simulink model "cantoni_combined_matrices_3pools_gates_experiment_splitting_combined"  (R2019b)
settings: Solver=FixedStepDiscrete  StartTime=0.0  StopTime=60*30  FixedStep=1  RelTol=1e-3
undefined symbols (not defined in the file or in its folder): comb_contr, comb_K, comb_plant_disc, comb_plant_disc_p, comb_plant_disc_w, ddelay, Pd, Pd0, Wd
settings Model: Creator=Jacob  LastModifiedBy=bas
settings DataIOCC: ReturnWorkspaceOutputs=off
settings SFSimCC: CustomCodeUndefinedFunction=UseInterfaceOnly

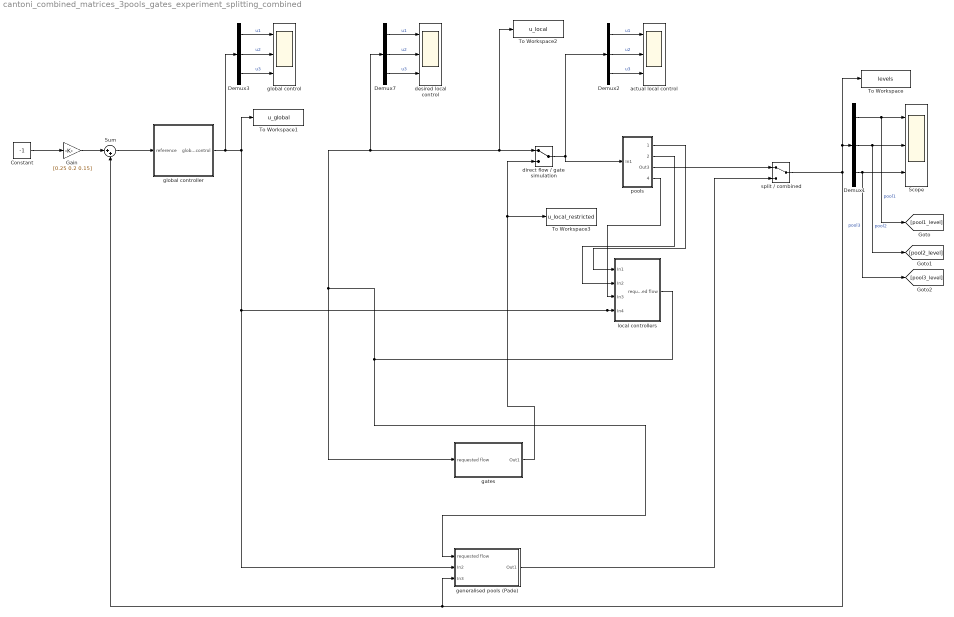
== system cantoni_combined_matrices_3pools_gates_experiment_splitting_combined ==
  Constant : Constant  Value=-1
  Demux{1..3,7} (4 alike) : Demux  Outputs=3
  Gain : Gain  Gain=[0.25 0.2 0.15]
  Scope : Scope  NumInputPorts=3
  Sum : Sum  Inputs=|++
  To Workspace : ToWorkspace  VariableName=levels  SaveFormat=Timeseries  SampleTime=-1
  To Workspace1 : ToWorkspace  VariableName=u_global  SaveFormat=Timeseries  SampleTime=-1
  To Workspace2 : ToWorkspace  VariableName=u_local  SaveFormat=Timeseries  SampleTime=-1
  To Workspace3 : ToWorkspace  VariableName=u_local_restricted  SaveFormat=Timeseries  SampleTime=-1
  actual local control : Scope  NumInputPorts=3
  desired local control : Scope  NumInputPorts=3
  direct flow / gate simulation : ManualSwitch
  gates : Subsystem
  generalised pools (Pade) : Subsystem
  global control : Scope  NumInputPorts=3
  global controller : Subsystem
  local controllers : Subsystem
  pools : Subsystem
  split / combined : ManualSwitch
  wires:
  Constant/1 -> Gain/1
  Gain/1 -> Sum/1
  split / combined/1 -> Sum/2, generalised pools (Pade)/3(In3), Demux1/1, To Workspace/1
  Demux1/1 -> Scope/1, [pool1_level]  "pool1"
  Demux1/2 -> [pool2_level], Scope/2  "pool2"
  Demux1/3 -> [pool3_level], Scope/3  "pool3"
  Demux3/3 -> global control/3  "u3"
  Demux3/2 -> global control/2  "u2"
  Demux3/1 -> global control/1  "u1"
  global controller/1(global_control) -> To Workspace1/1, local controllers/4(In4), generalised pools (Pade)/2(In2), Demux3/1
  Sum/1 -> global controller/1(reference)
  Demux2/3 -> actual local control/3  "u3"
  Demux2/1 -> actual local control/1  "u1"
  Demux2/2 -> actual local control/2  "u2"
  direct flow / gate simulation/1 -> Demux2/1, pools/1(In1)
  Demux7/3 -> desired local control/3  "u3"
  Demux7/2 -> desired local control/2  "u2"
  Demux7/1 -> desired local control/1  "u1"
  pools/3(Out3) -> split / combined/1
  gates/1(Out1) -> To Workspace3/1, direct flow / gate simulation/2
  generalised pools (Pade)/1(Out1) -> split / combined/2
  local controllers/1(requested flow) -> gates/1(requested flow), To Workspace2/1, direct flow / gate simulation/1, Demux7/1, generalised pools (Pade)/1(requested flow)
  pools/1(in_pool1) -> local controllers/1(In1)
  pools/2(in_pool2) -> local controllers/2(In2)
  pools/4(in_pool3) -> local controllers/3(In3)

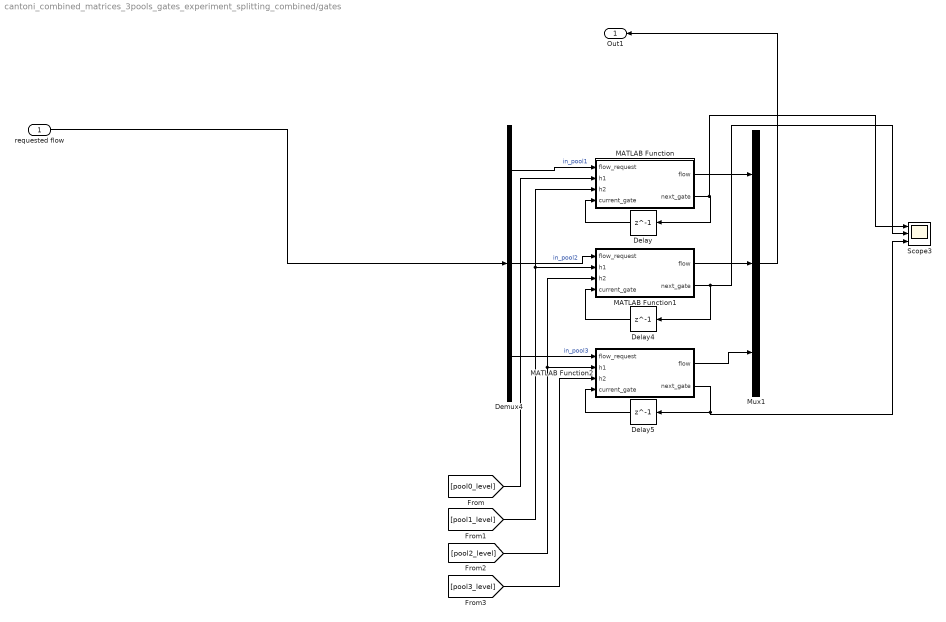
== system cantoni_combined_matrices_3pools_gates_experiment_splitting_combined/gates ==
  requested flow : Inport
  Delay : Delay  DelayLength=1
  Delay4 : Delay  DelayLength=1
  Delay5 : Delay  DelayLength=1
  Demux4 : Demux  Outputs=3
  MATLAB Function : MATLAB Function  TreatAsAtomicUnit=on
  MATLAB Function1 : MATLAB Function  TreatAsAtomicUnit=on
  MATLAB Function2 : MATLAB Function  TreatAsAtomicUnit=on
  Mux1 : Mux  Inputs=3
  Scope3 : Scope  NumInputPorts=3
  Out1 : Outport
  wires:
  Mux1/1 -> Out1/1
  requested flow/1 -> Demux4/1
  [pool2_level] -> MATLAB Function2/2(h1), MATLAB Function1/3(h2)
  Demux4/1 -> MATLAB Function/1(flow_request)  "in_pool1"
  Delay4/1 -> MATLAB Function1/4(current_gate)
  Delay5/1 -> MATLAB Function2/4(current_gate)
  Demux4/2 -> MATLAB Function1/1(flow_request)  "in_pool2"
  MATLAB Function1/2(next_gate) -> Scope3/2, Delay4/1
  [pool3_level] -> MATLAB Function2/3(h2)
  MATLAB Function1/1(flow) -> Mux1/2
  MATLAB Function2/1(flow) -> Mux1/3
  [pool1_level] -> MATLAB Function1/2(h1), MATLAB Function/3(h2)
  Delay/1 -> MATLAB Function/4(current_gate)
  MATLAB Function/1(flow) -> Mux1/1
  Demux4/3 -> MATLAB Function2/1(flow_request)  "in_pool3"
  [pool0_level] -> MATLAB Function/2(h1)
  MATLAB Function2/2(next_gate) -> Scope3/3, Delay5/1
  MATLAB Function/2(next_gate) -> Scope3/1, Delay/1

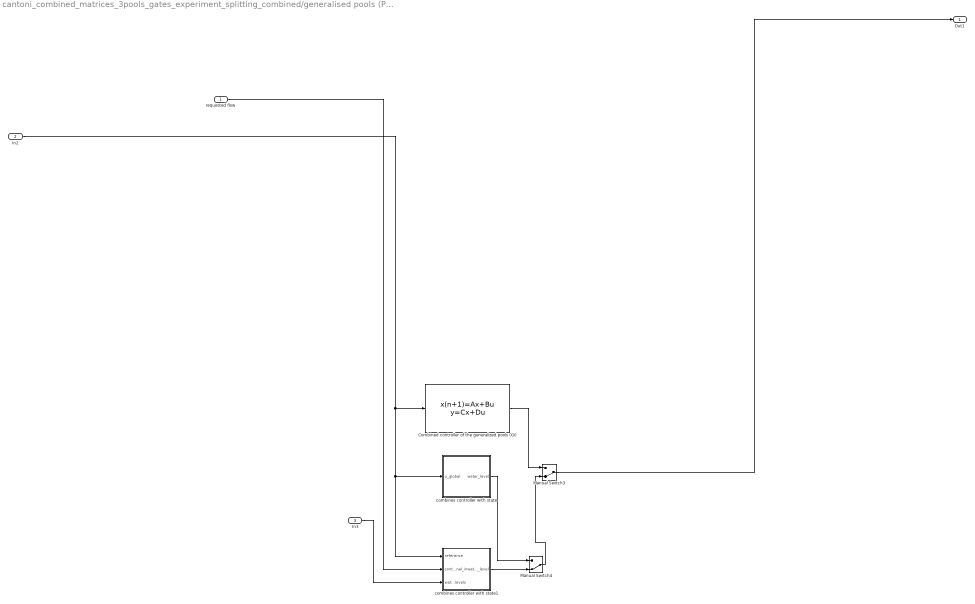
== system cantoni_combined_matrices_3pools_gates_experiment_splitting_combined/generalised pools (Pade) ==
  requested flow : Inport
  In2 : Inport  Port=2
  In3 : Inport  Port=3
  Combined controller of the generalized pools (Gi) : DiscreteStateSpace  A=comb_plant_disc.A  B=comb_plant_disc.B  C=comb_plant_disc.C  D=comb_plant_disc.D  SampleTime=-1
  Manual Switch3 : ManualSwitch  CurrentSetting=0
  Manual Switch4 : ManualSwitch  CurrentSetting=0
  combines controller with state : Subsystem
  combines controller with state1 : Subsystem
  Out1 : Outport
  wires:
  requested flow/1 -> combines controller with state1/2(control_signal_in)
  Combined controller of the generalized pools (Gi)/1 -> Manual Switch3/1
  Manual Switch4/1 -> Manual Switch3/2
  combines controller with state1/1(water_level) -> Manual Switch4/2
  Manual Switch3/1 -> Out1/1
  combines controller with state/1(water_level) -> Manual Switch4/1
  In3/1 -> combines controller with state1/3(water_levels)
  In2/1 -> combines controller with state1/1(reference), combines controller with state/1(u_global), Combined controller of the generalized pools (Gi)/1

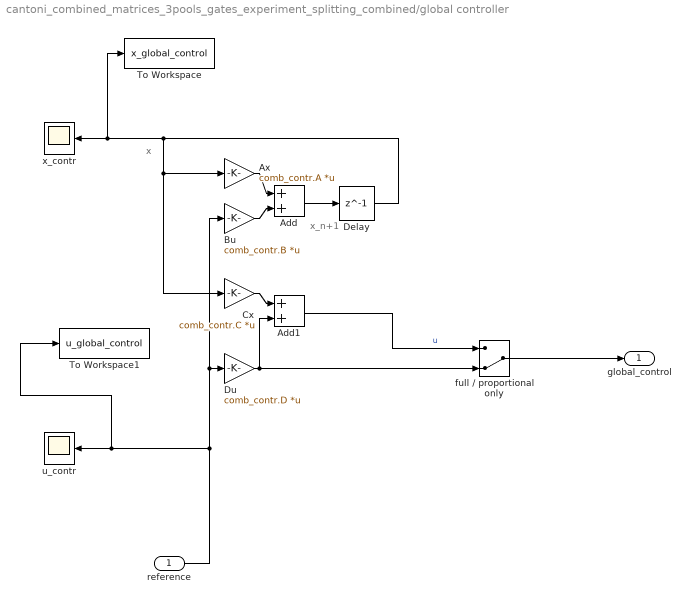
== system cantoni_combined_matrices_3pools_gates_experiment_splitting_combined/global controller ==
  note: x
  note: x_n+1
  reference : Inport
  Add : Sum
  Add1 : Sum
  Ax : Gain  Gain=comb_contr.A  Multiplication=Matrix(K*u)
  Bu : Gain  Gain=comb_contr.B  Multiplication=Matrix(K*u)
  Cx : Gain  Gain=comb_contr.C  Multiplication=Matrix(K*u)
  Delay : Delay  DelayLength=1  InitialCondition=[0;0;0;0;0;0;0;0;0;0;0;0;0;0;0]
  Du : Gain  Gain=comb_contr.D  Multiplication=Matrix(K*u)
  To Workspace : ToWorkspace  VariableName=x_global_control  SaveFormat=Timeseries  SampleTime=-1
  To Workspace1 : ToWorkspace  VariableName=u_global_control  SaveFormat=Timeseries  SampleTime=-1
  full / proportional only : ManualSwitch  CurrentSetting=0
  u_contr : Scope
  x_contr : Scope
  global_control : Outport
  wires:
  Bu/1 -> Add/2
  Cx/1 -> Add1/1
  Add/1 -> Delay/1
  Add1/1 -> full / proportional only/1  "u"
  Ax/1 -> Add/1
  Du/1 -> Add1/2, full / proportional only/2
  full / proportional only/1 -> global_control/1
  reference/1 -> Bu/1, Du/1, To Workspace1/1, u_contr/1
  Delay/1 -> To Workspace/1, x_contr/1, Cx/1, Ax/1

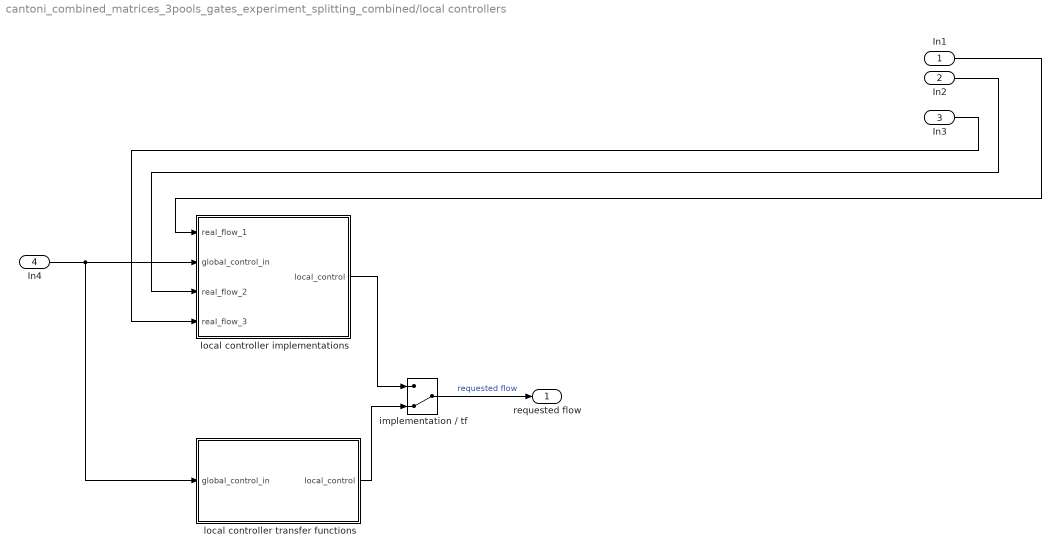
== system cantoni_combined_matrices_3pools_gates_experiment_splitting_combined/local controllers ==
  In1 : Inport
  In2 : Inport  Port=2
  In3 : Inport  Port=3
  In4 : Inport  Port=4
  implementation / tf : ManualSwitch  CurrentSetting=0
  local controller implementations : Subsystem
  local controller transfer functions : Subsystem
  requested flow : Outport
  wires:
  In2/1 -> local controller implementations/3(real_flow_2)
  In3/1 -> local controller implementations/4(real_flow_3)
  implementation / tf/1 -> requested flow/1  "requested flow"
  local controller transfer functions/1(local_control) -> implementation / tf/2
  In1/1 -> local controller implementations/1(real_flow_1)
  In4/1 -> local controller transfer functions/1(global_control_in), local controller implementations/2(global_control_in)
  local controller implementations/1(local_control) -> implementation / tf/1

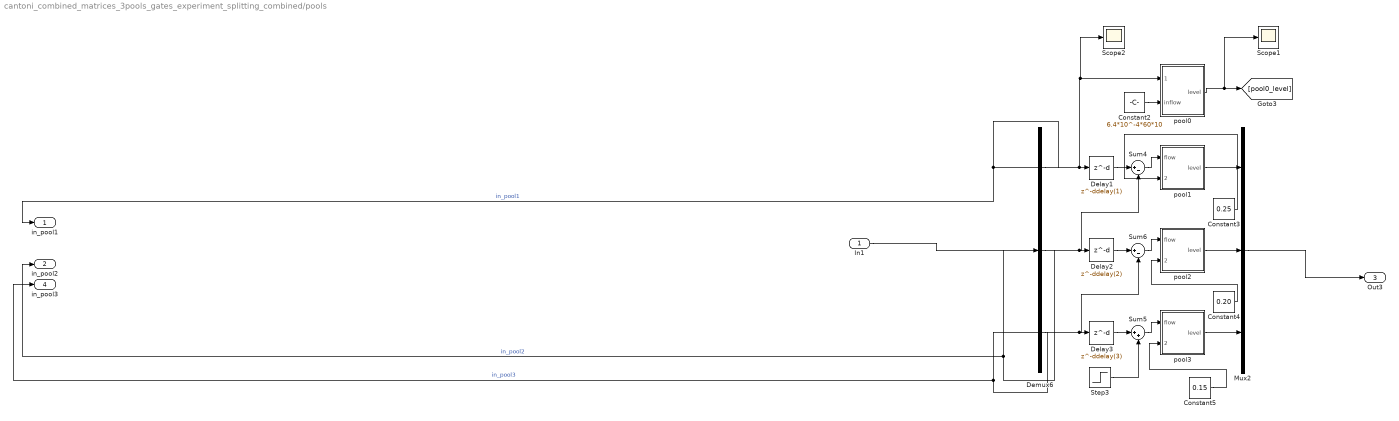
== system cantoni_combined_matrices_3pools_gates_experiment_splitting_combined/pools ==
  In1 : Inport
  Constant2 : Constant  Value=6.4*10^-4*60*10
  Constant3 : Constant  Value=0.25  SampleTime=-1
  Constant4 : Constant  Value=0.20
  Constant5 : Constant  Value=0.15
  Delay1 : Delay  DelayLength=ddelay(1)
  Delay2 : Delay  DelayLength=ddelay(2)
  Delay3 : Delay  DelayLength=ddelay(3)
  Demux6 : Demux  Outputs=3
  Mux2 : Mux  Inputs=3
  Scope1 : Scope
  Scope2 : Scope
  Step3 : Step  Time=100  After=-0.015  SampleTime=0
  Sum4 : Sum  Inputs=|+-
  Sum5 : Sum  Inputs=|++
  Sum6 : Sum  Inputs=|+-
  pool0 : Subsystem
  pool1 : Subsystem
  pool2 : Subsystem
  pool3 : Subsystem
  in_pool1 : Outport
  in_pool2 : Outport  Port=2
  Out3 : Outport  Port=3
  in_pool3 : Outport  Port=4
  wires:
  Mux2/1 -> Out3/1
  pool2/1(level) -> Mux2/2
  Sum6/1 -> pool2/1(flow)
  Sum4/1 -> pool1/1(flow)
  pool3/1(level) -> Mux2/3
  Delay3/1 -> Sum5/1
  pool1/1(level) -> Mux2/1
  Delay2/1 -> Sum6/1
  Delay1/1 -> Sum4/1
  Demux6/2 -> in_pool2/1, Sum4/2, Delay2/1  "in_pool2"
  Constant2/1 -> pool0/2(inflow)
  pool0/1(level) -> Scope1/1, [pool0_level]
  Sum5/1 -> pool3/1(flow)
  Step3/1 -> Sum5/2
  In1/1 -> Demux6/1
  Constant3/1 -> pool1/2("initial_level ")
  Demux6/3 -> in_pool3/1, Sum6/2, Delay3/1  "in_pool3"
  Constant4/1 -> pool2/2(initial_level)
  Constant5/1 -> pool3/2(initial_level)
  Demux6/1 -> in_pool1/1, Scope2/1, pool0/1(outflow), Delay1/1  "in_pool1"

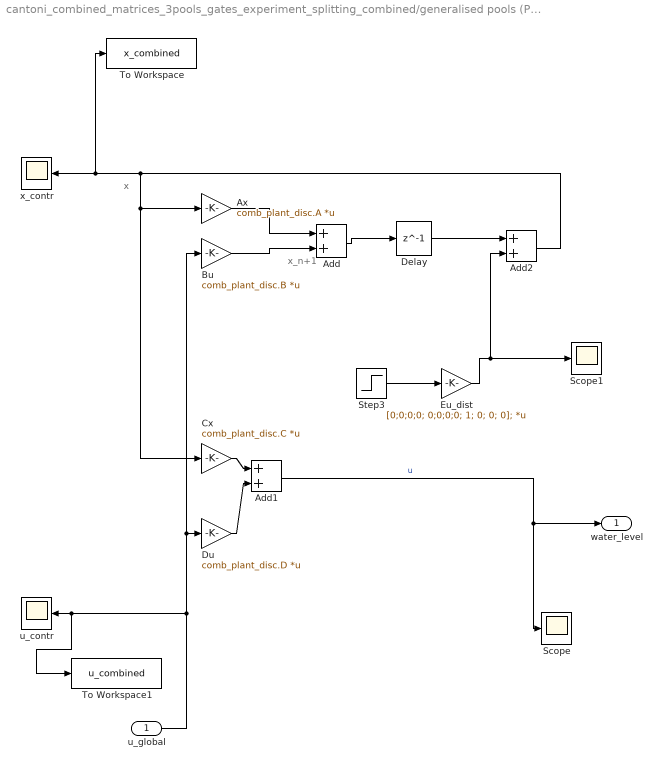
== system cantoni_combined_matrices_3pools_gates_experiment_splitting_combined/generalised pools (Pade)/combines controller with state ==
  note: x
  note: x_n+1
  u_global : Inport
  Add : Sum
  Add1 : Sum
  Add2 : Sum
  Ax : Gain  Gain=comb_plant_disc.A  Multiplication=Matrix(K*u)
  Bu : Gain  Gain=comb_plant_disc.B  Multiplication=Matrix(K*u)
  Cx : Gain  Gain=comb_plant_disc.C  Multiplication=Matrix(K*u)
  Delay : Delay  DelayLength=1  InitialCondition=[0.25;0;0;0;0.20;0;0;0;0.15;0;0;0]
  Du : Gain  Gain=comb_plant_disc.D  Multiplication=Matrix(K*u)
  Eu_dist : Gain  Gain=[0;0;0;0; 0;0;0;0; 1; 0; 0; 0];  Multiplication=Matrix(K*u)
  Scope : Scope
  Scope1 : Scope
  Step3 : Step  Time=100  After=-0.015/0.2279* 1/60  SampleTime=0
  To Workspace : ToWorkspace  VariableName=x_combined  SaveFormat=Timeseries  SampleTime=-1
  To Workspace1 : ToWorkspace  VariableName=u_combined  SaveFormat=Timeseries  SampleTime=-1
  u_contr : Scope
  x_contr : Scope
  water_level : Outport
  wires:
  Bu/1 -> Add/2
  Cx/1 -> Add1/1
  Add/1 -> Delay/1
  Add1/1 -> water_level/1, Scope/1  "u"
  Ax/1 -> Add/1
  Du/1 -> Add1/2
  Add2/1 -> To Workspace/1, x_contr/1, Cx/1, Ax/1
  u_global/1 -> Bu/1, Du/1, To Workspace1/1, u_contr/1
  Step3/1 -> Eu_dist/1
  Eu_dist/1 -> Add2/2, Scope1/1
  Delay/1 -> Add2/1

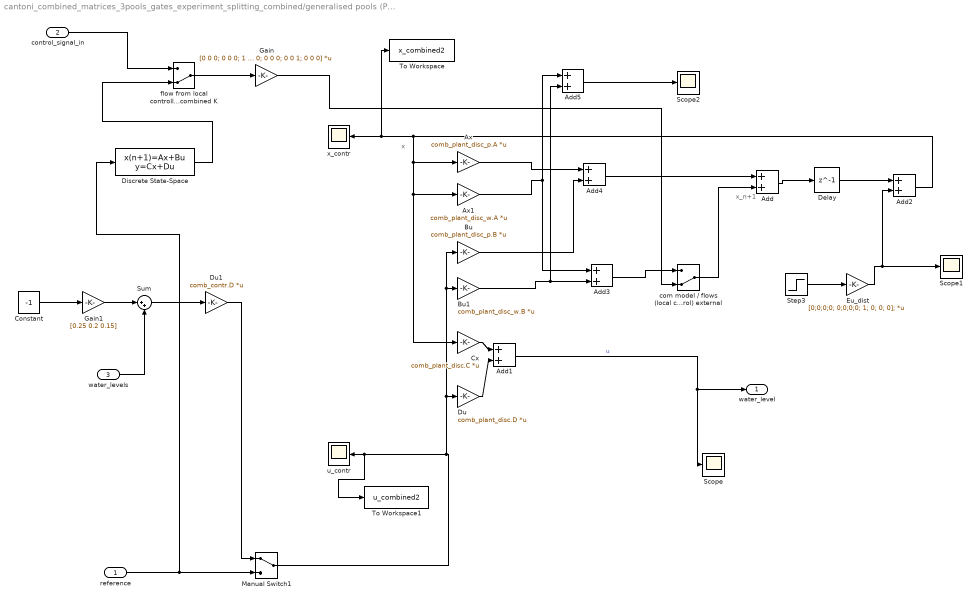
== system cantoni_combined_matrices_3pools_gates_experiment_splitting_combined/generalised pools (Pade)/combines controller with state1 ==
  note: x
  note: x_n+1
  reference : Inport
  control_signal_in : Inport  Port=2
  water_levels : Inport  Port=3
  Add{,1..5} (6 alike) : Sum
  Ax : Gain  Gain=comb_plant_disc_p.A  Multiplication=Matrix(K*u)
  Ax1 : Gain  Gain=comb_plant_disc_w.A  Multiplication=Matrix(K*u)
  Bu : Gain  Gain=comb_plant_disc_p.B  Multiplication=Matrix(K*u)
  Bu1 : Gain  Gain=comb_plant_disc_w.B  Multiplication=Matrix(K*u)
  Constant : Constant  Value=-1
  Cx : Gain  Gain=comb_plant_disc.C  Multiplication=Matrix(K*u)
  Delay : Delay  DelayLength=1  InitialCondition=[0.25;0;0;0;0.20;0;0;0;0.15;0;0;0]
  Discrete State-Space : DiscreteStateSpace  A=comb_K.A  B=comb_K.B  C=comb_K.C  D=comb_K.D  SampleTime=-1
  Du : Gain  Gain=comb_plant_disc.D  Multiplication=Matrix(K*u)
  Du1 : Gain  Gain=comb_contr.D  Multiplication=Matrix(K*u)
  Eu_dist : Gain  Gain=[0;0;0;0; 0;0;0;0; 1; 0; 0; 0];  Multiplication=Matrix(K*u)
  Gain : Gain  Gain=[0 0 0; 0 0 0; 1 0 0; 0 0 0; 0 0 0; 0 0 0; 0 1 0; 0 0 0; 0 0 0; 0 0 0; 0 0 1; 0 0 0]  Multiplication=Matrix(K*u)
  Gain1 : Gain  Gain=[0.25 0.2 0.15]
  Manual Switch1 : ManualSwitch
  Scope : Scope
  Scope1 : Scope
  Scope2 : Scope
  Step3 : Step  Time=100  After=-0.015/0.2279* 1/60  SampleTime=0
  Sum : Sum  Inputs=|++
  To Workspace : ToWorkspace  VariableName=x_combined2  SaveFormat=Timeseries  SampleTime=-1
  To Workspace1 : ToWorkspace  VariableName=u_combined2  SaveFormat=Timeseries  SampleTime=-1
  com model / flows (local control) external : ManualSwitch  CurrentSetting=0
  flow from local controllers / flow from combined K : ManualSwitch  CurrentSetting=0
  u_contr : Scope
  x_contr : Scope
  water_level : Outport
  wires:
  Cx/1 -> Add1/1
  Add/1 -> Delay/1
  Add1/1 -> water_level/1, Scope/1  "u"
  Du/1 -> Add1/2
  Add2/1 -> To Workspace/1, x_contr/1, Ax1/1, Cx/1, Ax/1
  Manual Switch1/1 -> u_contr/1, To Workspace1/1, Bu1/1, Bu/1, Du/1
  Step3/1 -> Eu_dist/1
  Eu_dist/1 -> Add2/2, Scope1/1
  Delay/1 -> Add2/1
  Add4/1 -> Add/1
  Ax/1 -> Add4/1
  Ax1/1 -> Add3/1, Add5/1
  Bu/1 -> Add4/2
  Bu1/1 -> Add5/2, Add3/2
  Add5/1 -> Scope2/1
  control_signal_in/1 -> flow from local controllers / flow from combined K/1
  com model / flows (local control) external/1 -> Add/2
  Add3/1 -> com model / flows (local control) external/1
  Gain/1 -> com model / flows (local control) external/2
  water_levels/1 -> Sum/2
  reference/1 -> Discrete State-Space/1, Manual Switch1/2
  Du1/1 -> Manual Switch1/1
  Gain1/1 -> Sum/1
  Constant/1 -> Gain1/1
  Sum/1 -> Du1/1
  Discrete State-Space/1 -> flow from local controllers / flow from combined K/2
  flow from local controllers / flow from combined K/1 -> Gain/1

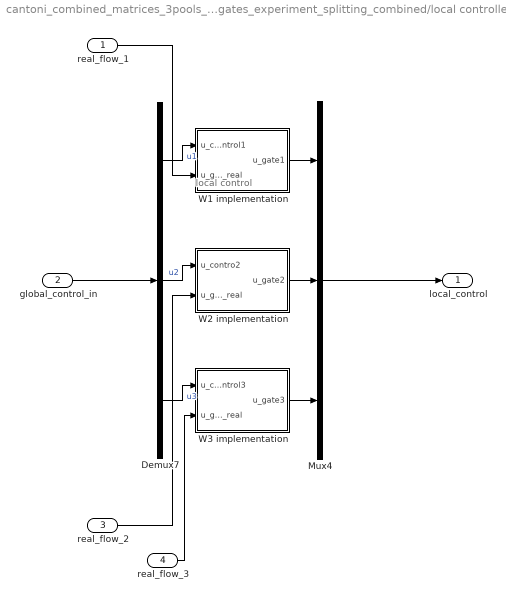
== system cantoni_combined_matrices_3pools_gates_experiment_splitting_combined/local controllers/local controller implementations ==
  note: local control
  real_flow_1 : Inport
  global_control_in : Inport  Port=2
  real_flow_2 : Inport  Port=3
  real_flow_3 : Inport  Port=4
  Demux7 : Demux  Outputs=3
  Mux4 : Mux  Inputs=3
  W1 implementation : Subsystem
  W2 implementation : Subsystem
  W3 implementation : Subsystem
  local_control : Outport
  wires:
  Demux7/1 -> W1 implementation/1(u_control1)  "u1"
  W1 implementation/1(u_gate1) -> Mux4/1
  Demux7/3 -> W3 implementation/1(u_control3)  "u3"
  real_flow_3/1 -> W3 implementation/2(u_gate3_real)
  real_flow_2/1 -> W2 implementation/2(u_gate2_real)
  Demux7/2 -> W2 implementation/1(u_contro2)  "u2"
  global_control_in/1 -> Demux7/1
  Mux4/1 -> local_control/1
  W3 implementation/1(u_gate3) -> Mux4/3
  real_flow_1/1 -> W1 implementation/2(u_gate1_real)
  W2 implementation/1(u_gate2) -> Mux4/2

== system cantoni_combined_matrices_3pools_gates_experiment_splitting_combined/local controllers/local controller transfer functions ==
  global_control_in : Inport
  Demux4 : Demux  Outputs=3
  Mux3 : Mux  Inputs=3
  W1 : DiscreteTransferFcn  Numerator=Wd{1}.Numerator{1}  Denominator=Wd{1}.Denominator{1}
  W2 : DiscreteTransferFcn  Numerator=Wd{2}.Numerator{1}  Denominator=Wd{2}.Denominator{1}
  W3 : DiscreteTransferFcn  Numerator=Wd{3}.Numerator{1}  Denominator=Wd{3}.Denominator{1}
  local_control : Outport
  wires:
  Mux3/1 -> local_control/1
  global_control_in/1 -> Demux4/1
  Demux4/3 -> W3/1  "u3"
  W3/1 -> Mux3/3
  Demux4/2 -> W2/1  "u2"
  W2/1 -> Mux3/2
  W1/1 -> Mux3/1
  Demux4/1 -> W1/1  "u1"

== system cantoni_combined_matrices_3pools_gates_experiment_splitting_combined/pools/pool0 ==
  note: //TODO: remove overflow from pool
  outflow : Inport
  inflow : Inport  Port=2
  Add : Sum  Inputs=-+
  Constant : Constant  Value=0
  Saturation : Saturate  UpperLimit=0.3
  pool1 : DiscreteTransferFcn  Numerator=Pd0.Numerator{1}  Denominator=Pd0.Denominator{1}  InitialStatesSource=Input port
      settings: InputPortMap=u0,p5
  level : Outport
  wires:
  pool1/1 -> Saturation/1
  outflow/1 -> Add/1
  inflow/1 -> Add/2
  Add/1 -> pool1/1
  Constant/1 -> pool1/2
  Saturation/1 -> level/1

== system cantoni_combined_matrices_3pools_gates_experiment_splitting_combined/pools/pool1 ==
  flow : Inport
  "initial_level " : Inport  Port=2
  Gain : Gain  Gain=1/Pd{1}.Numerator{1}(2)
  P1 : DiscreteTransferFcn  Numerator=Pd{1}.Numerator{1}  Denominator=Pd{1}.Denominator{1}  InitialStatesSource=Input port
      settings: InputPortMap=u0,p5
  level : Outport
  wires:
  flow/1 -> P1/1
  P1/1 -> level/1
  Gain/1 -> P1/2
  "initial_level "/1 -> Gain/1

== system cantoni_combined_matrices_3pools_gates_experiment_splitting_combined/pools/pool2 ==
  flow : Inport
  initial_level : Inport  Port=2
  Gain : Gain  Gain=1/Pd{2}.Numerator{1}(2)
  P2 : DiscreteTransferFcn  Numerator=Pd{2}.Numerator{1}  Denominator=Pd{2}.Denominator{1}  InitialStatesSource=Input port
      settings: InputPortMap=u0,p5
  level : Outport
  wires:
  flow/1 -> P2/1
  P2/1 -> level/1
  Gain/1 -> P2/2
  initial_level/1 -> Gain/1

== system cantoni_combined_matrices_3pools_gates_experiment_splitting_combined/pools/pool3 ==
  flow : Inport
  initial_level : Inport  Port=2
  Gain : Gain  Gain=1/Pd{3}.Numerator{1}(2)
  P3 : DiscreteTransferFcn  Numerator=Pd{3}.Numerator{1}  Denominator=Pd{3}.Denominator{1}  InitialStatesSource=Input port
      settings: InputPortMap=u0,p5
  level : Outport
  wires:
  P3/1 -> level/1
  flow/1 -> P3/1
  Gain/1 -> P3/2
  initial_level/1 -> Gain/1

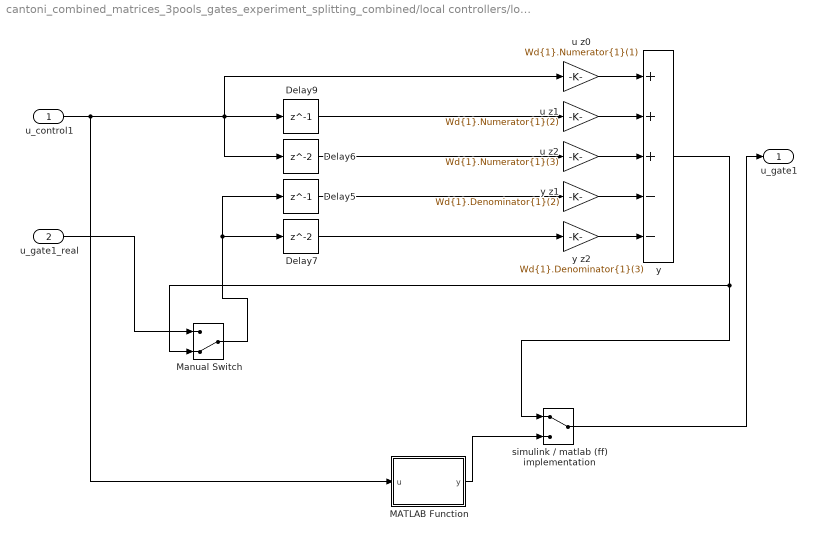
== system cantoni_combined_matrices_3pools_gates_experiment_splitting_combined/local controllers/local controller implementations/W1 implementation ==
  u_control1 : Inport
  u_gate1_real : Inport  Port=2
  Delay5 : Delay  DelayLength=1
  Delay6 : Delay
  Delay7 : Delay
  Delay9 : Delay  DelayLength=1
  MATLAB Function : MATLAB Function  TreatAsAtomicUnit=on
  Manual Switch : ManualSwitch  CurrentSetting=0
  simulink / matlab (ff) implementation : ManualSwitch
  u z0 : Gain  Gain=Wd{1}.Numerator{1}(1)
  u z1 : Gain  Gain=Wd{1}.Numerator{1}(2)
  u z2 : Gain  Gain=Wd{1}.Numerator{1}(3)
  y : Sum  Inputs=+++--
  y z1 : Gain  Gain=Wd{1}.Denominator{1}(2)
  y z2 : Gain  Gain=Wd{1}.Denominator{1}(3)
  u_gate1 : Outport
  wires:
  y z2/1 -> y/5
  Delay6/1 -> u z2/1
  y z1/1 -> y/4
  Delay7/1 -> y z2/1
  u z1/1 -> y/2
  u z2/1 -> y/3
  y/1 -> simulink / matlab (ff) implementation/1, Manual Switch/2
  Delay5/1 -> y z1/1
  u_control1/1 -> MATLAB Function/1(u), Delay6/1, u z0/1, Delay9/1
  u z0/1 -> y/1
  Delay9/1 -> u z1/1
  Manual Switch/1 -> Delay5/1, Delay7/1
  u_gate1_real/1 -> Manual Switch/1
  MATLAB Function/1(y) -> simulink / matlab (ff) implementation/2
  simulink / matlab (ff) implementation/1 -> u_gate1/1

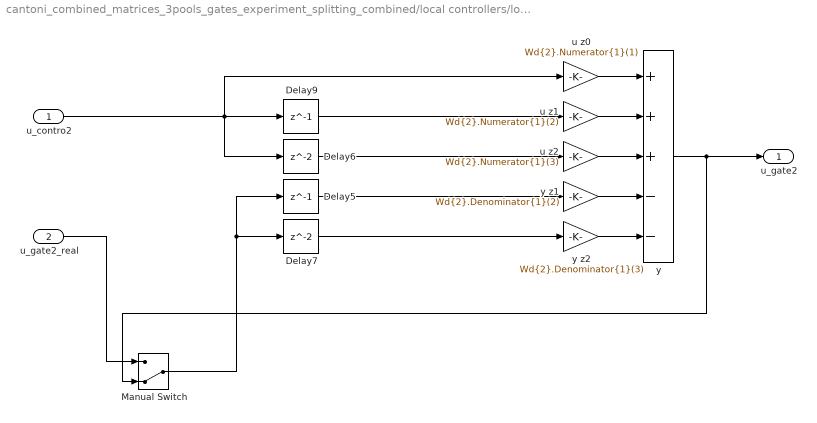
== system cantoni_combined_matrices_3pools_gates_experiment_splitting_combined/local controllers/local controller implementations/W2 implementation ==
  u_contro2 : Inport
  u_gate2_real : Inport  Port=2
  Delay5 : Delay  DelayLength=1
  Delay6 : Delay
  Delay7 : Delay
  Delay9 : Delay  DelayLength=1
  Manual Switch : ManualSwitch  CurrentSetting=0
  u z0 : Gain  Gain=Wd{2}.Numerator{1}(1)
  u z1 : Gain  Gain=Wd{2}.Numerator{1}(2)
  u z2 : Gain  Gain=Wd{2}.Numerator{1}(3)
  y : Sum  Inputs=+++--
  y z1 : Gain  Gain=Wd{2}.Denominator{1}(2)
  y z2 : Gain  Gain=Wd{2}.Denominator{1}(3)
  u_gate2 : Outport
  wires:
  y z2/1 -> y/5
  Delay6/1 -> u z2/1
  y z1/1 -> y/4
  Delay7/1 -> y z2/1
  u z1/1 -> y/2
  u z2/1 -> y/3
  y/1 -> Manual Switch/2, u_gate2/1
  Delay5/1 -> y z1/1
  u_contro2/1 -> Delay6/1, u z0/1, Delay9/1
  u z0/1 -> y/1
  Delay9/1 -> u z1/1
  Manual Switch/1 -> Delay5/1, Delay7/1
  u_gate2_real/1 -> Manual Switch/1

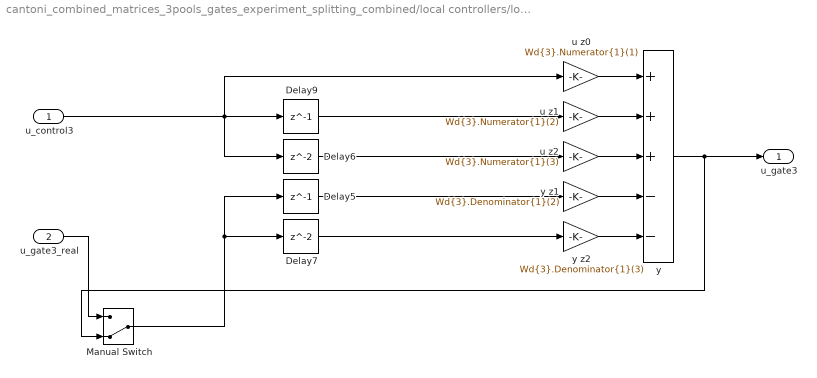
== system cantoni_combined_matrices_3pools_gates_experiment_splitting_combined/local controllers/local controller implementations/W3 implementation ==
  u_control3 : Inport
  u_gate3_real : Inport  Port=2
  Delay5 : Delay  DelayLength=1
  Delay6 : Delay
  Delay7 : Delay
  Delay9 : Delay  DelayLength=1
  Manual Switch : ManualSwitch  CurrentSetting=0
  u z0 : Gain  Gain=Wd{3}.Numerator{1}(1)
  u z1 : Gain  Gain=Wd{3}.Numerator{1}(2)
  u z2 : Gain  Gain=Wd{3}.Numerator{1}(3)
  y : Sum  Inputs=+++--
  y z1 : Gain  Gain=Wd{3}.Denominator{1}(2)
  y z2 : Gain  Gain=Wd{3}.Denominator{1}(3)
  u_gate3 : Outport
  wires:
  y z2/1 -> y/5
  Delay6/1 -> u z2/1
  y z1/1 -> y/4
  Delay7/1 -> y z2/1
  u z1/1 -> y/2
  u z2/1 -> y/3
  y/1 -> Manual Switch/2, u_gate3/1
  Delay5/1 -> y z1/1
  u_control3/1 -> Delay6/1, u z0/1, Delay9/1
  u z0/1 -> y/1
  Delay9/1 -> u z1/1
  Manual Switch/1 -> Delay5/1, Delay7/1
  u_gate3_real/1 -> Manual Switch/1

== matlab function cantoni_combined_matrices_3pools_gates_experiment_splitting_combined/gates/MATLAB Function1 ==
  data: flow_request input; flow output; h1 input; h2 input; current_gate input; next_gate output
function [flow, next_gate] = fcn(flow_request, h1, h2, current_gate)

[flow, next_gate] = gate_simulation(flow_request, h1, h2, current_gate);

== matlab function cantoni_combined_matrices_3pools_gates_experiment_splitting_combined/gates/MATLAB Function ==
  data: flow_request input; flow output; h1 input; h2 input; current_gate input; next_gate output
function [flow, next_gate] = fcn(flow_request, h1, h2, current_gate)

[flow, next_gate] = gate_simulation(flow_request, h1, h2, current_gate);

== matlab function cantoni_combined_matrices_3pools_gates_experiment_splitting_combined/gates/MATLAB Function2 ==
  data: flow_request input; flow output; h1 input; h2 input; current_gate input; next_gate output
function [flow, next_gate] = fcn(flow_request, h1, h2, current_gate)

[flow, next_gate] = gate_simulation(flow_request, h1, h2, current_gate);

== matlab function cantoni_combined_matrices_3pools_gates_experiment_splitting_combined/local controllers/local controller implementations/W1 implementation/MATLAB Function ==
  data: u input; y output
function y = fcn(u)

persistent y_z1;
persistent y_z0;
persistent u_z1;
persistent u_z0;

if isempty(y_z1)
 y_z1 = 0;
 y_z0 = 0;
 u_z1 = 0;
 u_z0 = 0;
end


ku0 = 1.539744e-01;
ku1 = 2.564103e-04;
ku2 = -1.537179e-01;
ky1 = -1.846154e+00;
ky2 = 8.461538e-01;
    %// calculate y
y = ku0 * u + ku1 * u_z0 + ku2 * u_z1 - ky1 * y_z0 - ky2 * y_z1;

    %// update delays
    y_z1 = y_z0;
    y_z0 = y; %// not useful anymore due to ant-wind-up scheme
    u_z1 = u_z0;
    u_z0 = u; %// not useful anymore due to ant-wind-up scheme



% static double ku0[NUM_ACTUATORS] = {1.539744e-01, 2.309615e-01, 1.539744e-01};
% static double ku1[NUM_ACTUATORS] = {2.564103e-04, 3.846154e-04, 2.564103e-04};
% static double ku2[NUM_ACTUATORS] = {-1.537179e-01, -2.305769e-01, -1.537179e-01};
% static double ky1[NUM_ACTUATORS] = {-1.846154e+00, -1.846154e+00, -1.846154e+00};
% static double ky2[NUM_ACTUATORS] = {8.461538e-01, 8.461538e-01, 8.461538e-01};
